simulink model "prob_1"  (R2015a)
settings: Solver=ode45  StartTime=0.0  StopTime=10.0  RelTol=1e-3
settings Model: Creator=Anu  LastModifiedBy=Anu

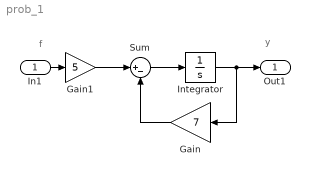
== system prob_1 ==
  note: y
  note: f
  In1 : Inport
  Gain : Gain  Gain=7
  Gain1 : Gain  Gain=5
  Integrator : Integrator
  Sum : Sum  Inputs=|+-
  Out1 : Outport
  wires:
  Gain1/1 -> Sum/1
  Sum/1 -> Integrator/1
  Integrator/1 -> Gain/1, Out1/1
  Gain/1 -> Sum/2
  In1/1 -> Gain1/1
